simulink model "Delete"  (R2020b)
settings: Solver=VariableStepAuto  StartTime=0.0  StopTime=10.0  RelTol=1e-3
libraries: simulink_extras x4, pid_lib x1
settings Model: Creator=ndroz  LastModifiedBy=ndroz

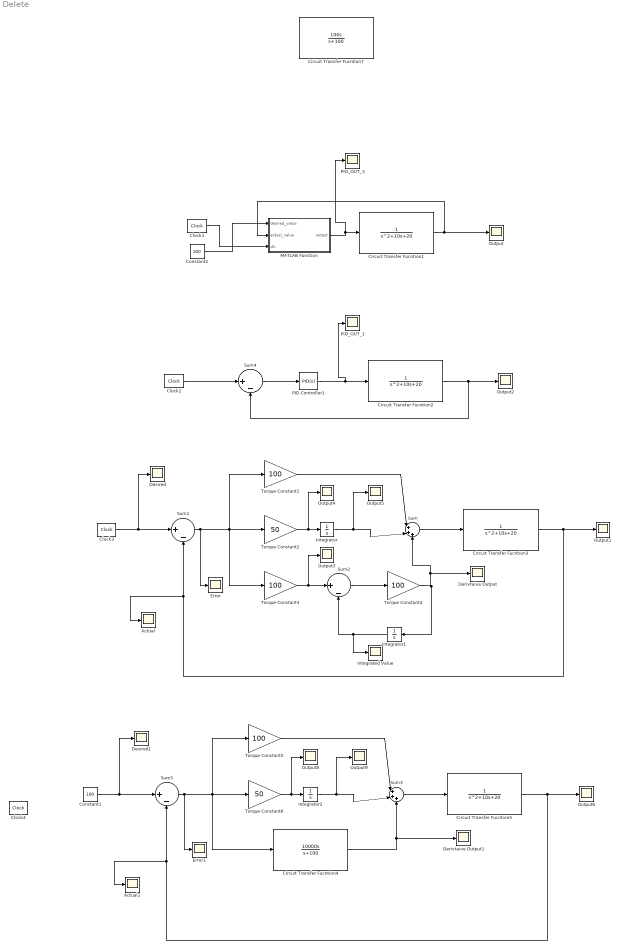
== system Delete ==
  Actual : Scope
  Actual1 : Scope
  Circuit Transfer Fucntion{1..3,5} (4 alike) : TransferFcn  Denominator=[1 10 20]
  Circuit Transfer Fucntion4 : TransferFcn  Numerator=[10000 0]  Denominator=[1 100]
  Circuit Transfer Fucntion7 : TransferFcn  Numerator=[100 0]  Denominator=[1 100]
  Clock{1..4} (4 alike) : simulink_extras/Flip Flops/Clock  period=0.01
  Constant1 : Constant  Value=100
  Constant2 : Constant  Value=100
  Derivtaive Output : Scope
  Derivtaive Output1 : Scope
  Desired : Scope
  Desired1 : Scope
  Error : Scope
  Error1 : Scope
  Integrated Value : Scope
  Integrator : Integrator
  Integrator1 : Integrator
  Integrator2 : Integrator
  MATLAB Function : MATLAB Function  TreatAsAtomicUnit=on
  Output{,1..6,8..9} (9 alike) : Scope
  PID Controller1 : pid_lib/PID Controller  Controller=PID  Form=Parallel  TimeDomain=Continuous-time  UseExternalTs=off  SampleTime=-1  IntegratorMethod=Forward Euler  FilterMethod=Forward Euler  ControllerParametersSource=internal  P=100  I=50  D=100  UseFilter=on  N=100  TunerSelectOption=Transfer Function Based (PID Tuner App)  InitialConditionSource=internal  InitialConditionForIntegrator=0  InitialConditionForFilter=0  DifferentiatorICPrevScaledInput=0  ExternalReset=none  TrackingMode=off  Kt=1  LimitOutput=off  SatLimitsSource=internal  UpperSaturationLimit=inf  LowerSaturationLimit=-inf  LinearizeAsGain=on  AntiWindupMode=none  Kb=1  POutMin=[]  POutMax=[]  IOutMin=[]  IOutMax=[]  DOutMin=[]  DOutMax=[]  NOutMin=[]  NOutMax=[]  SumOutMin=[]  SumOutMax=[]  SaturationOutMin=[]  SaturationOutMax=[]  PParamMin=[]  PParamMax=[]  IParamMin=[]  IParamMax=[]  DParamMin=[]  DParamMax=[]  NParamMin=[]  NParamMax=[]  KbParamMin=[]  KbParamMax=[]  KtParamMin=[]  KtParamMax=[]  KbOutMin=[]  KbOutMax=[]  KtOutMin=[]  KtOutMax=[]  IntegratorOutMin=[]  IntegratorOutMax=[]  FilterOutMin=[]  FilterOutMax=[]  SumI1OutMin=[]  SumI1OutMax=[]  SumI2OutMin=[]  SumI2OutMax=[]  SumI3OutMin=[]  SumI3OutMax=[]  SumI4OutMin=[]  SumI4OutMax=[]  SumDOutMin=[]  SumDOutMax=[]  DifferentiatorOutMin=[]  DifferentiatorOutMax=[]  FilterDiffOutCoefMin=[]  FilterDiffOutCoefMax=[]  ReciprocalOutMin=[]  ReciprocalOutMax=[]  SumDenOutMin=[]  SumDenOutMax=[]  SumNumOutMin=[]  SumNumOutMax=[]  DivideOutMin=[]  DivideOutMax=[]  UdiffTsProdOutMin=[]  UdiffTsProdOutMax=[]  NTsProdOutMin=[]  NTsProdOutMax=[]  UintegralTsProdOutMin=[]  UintegralTsProdOutMax=[]  UngainTsProdOutMin=[]  UngainTsProdOutMax=[]  IntegratorContinuousStateAttributes=''  IntegratorStateMustResolveToSignalObject=off  IntegratorRTWStateStorageClass=Auto  FilterContinuousStateAttributes=''  FilterStateMustResolveToSignalObject=off  FilterRTWStateStorageClass=Auto  ParallelPVariant=InternalParameters  IdealPVariant=Disabled  IVariant=InternalParameters  DVariant=InternalParameters  IntegratorVariant=Continuous  SatVariant=Disabled  AWVariant=Passthrough  PCopyVariant=Disabled  TRVariant=Disabled  FdbkBlocksVariant=Forward  IdealPFdbkVariant=Disabled  SatFdbkVariant=Disabled  DerivativeFilterVariant=ContFilter  NVariant=InternalParameters  NCopyVariant=Disabled  FilterICVariant=InternalICsFilter  IntegratorICVariant=InternalICs  ExternalResetVariant=Disabled  TRSumVariant=Passthrough  SumFdbkVariant=Disabled  SumVariant=Sum_PID  TsampFilterVariant=InternalTs  TsampNgainVariant=Passthrough  TsampIntegralVariant=Passthrough  ExternalSaturationOutDataTypeStr=Inherit: Same as second input
  PID_OUT_1 : Scope
  PID_OUT_3 : Scope
  Sum : Sum  Inputs=|+++
  Sum{1..2,4..5} (4 alike) : Sum  Inputs=|+-
  Sum3 : Sum  Inputs=|+++
  Torque Constant{1,3..5} (4 alike) : Gain  Gain=100
  Torque Constant2 : Gain  Gain=50
  Torque Constant6 : Gain  Gain=50
  wires:
  MATLAB Function/1(output) -> PID_OUT_3/1, Circuit Transfer Fucntion1/1
  Circuit Transfer Fucntion1/1 -> MATLAB Function/2(actual_value), Output/1
  Circuit Transfer Fucntion2/1 -> Output2/1, Sum4/2
  Clock2/1 -> Sum4/1
  Sum4/1 -> PID Controller1/1
  PID Controller1/1 -> PID_OUT_1/1, Circuit Transfer Fucntion2/1
  Circuit Transfer Fucntion3/1 -> Actual/1, Sum1/2, Output1/1
  Clock3/1 -> Desired/1, Sum1/1
  Sum1/1 -> Error/1, Torque Constant3/1, Torque Constant2/1, Torque Constant1/1
  Torque Constant1/1 -> Sum/1
  Torque Constant2/1 -> Output4/1, Integrator/1
  Integrator/1 -> Output5/1, Sum/2
  Torque Constant3/1 -> Output3/1, Sum2/1
  Sum2/1 -> Torque Constant4/1
  Torque Constant4/1 -> Sum/3, Derivtaive Output/1, Integrator1/1
  Integrator1/1 -> Integrated Value/1, Sum2/2
  Sum/1 -> Circuit Transfer Fucntion3/1
  Torque Constant6/1 -> Output8/1, Integrator2/1
  Sum3/1 -> Circuit Transfer Fucntion5/1
  Integrator2/1 -> Output9/1, Sum3/2
  Circuit Transfer Fucntion5/1 -> Actual1/1, Sum5/2, Output6/1
  Torque Constant5/1 -> Sum3/1
  Circuit Transfer Fucntion4/1 -> Derivtaive Output1/1, Sum3/3
  Sum5/1 -> Error1/1, Circuit Transfer Fucntion4/1, Torque Constant6/1, Torque Constant5/1
  Constant1/1 -> Desired1/1, Sum5/1
  Constant2/1 -> MATLAB Function/1(desired_value)
  Clock1/1 -> MATLAB Function/3(clk)

== matlab function Delete/MATLAB Function ==
  settings: updateMethod=DISCRETE
  data: desired_value input; output output; actual_value input; clk input
function output = PID(desired_value, actual_value, clk)
    persistent pid_integrator pid_prev_error pid_lim_min pid_lim_max pid_lim_min_int pid_lim_max_int sample_time Kp Ki Kd Tau diff_array diff_mult proportional pid_differentiator
    if isempty(pid_integrator)
        pid_integrator = 0;
        pid_prev_error = 0;
        pid_lim_min = -1000000;
        pid_lim_max = 1000000;
        pid_lim_min_int = -500;
        pid_lim_max_int = 500;
        sample_time = 0.01;
        Kp = 0;
        Ki = 0;
        Kd = 100;
        Tau = 100;
        diff_array = zeros(1,4);
        diff_mult = [exp(-Tau)^(7*sample_time/2) exp(-Tau)^(5*sample_time/2) exp(-Tau)^(3*sample_time/2) exp(-Tau)^(sample_time/2)];
        proportional = 0;
        pid_differentiator = 0;
    end
    
    if clk == 1
        error = desired_value - actual_value;

        %Proportional
        proportional = Kp*error;

        %Integral
        pid_integrator = pid_integrator + 0.5*Ki*sample_time*(error + pid_prev_error);

        if pid_integrator > pid_lim_max_int
            pid_integrator = pid_lim_max_int;
        elseif pid_integrator < pid_lim_min_int
            pid_integrator = pid_lim_min_int;
        end

        %Derivative
        %pid_differentiator = -(2*Kd*(actual_value - pid_prev_measurment) + (2*Tau - sample_time)*pid_differentiator) / (2*Tau + sample_time);
        diff_array(4) = Kd*(error - pid_prev_error)/sample_time;
        pid_differentiator = 0;
        for i = 1:length(diff_array)
           pid_differentiator = pid_differentiator + (diff_array(i)*diff_mult(i));
        end

        diff_array = circshift(diff_array,[0, -1]);
        pid_prev_error = error; 
    end
    
    output = proportional + pid_integrator + pid_differentiator;
    if output > pid_lim_max
       output = pid_lim_max;
    elseif output < pid_lim_min
       output = pid_lim_min;
    end
end
